simulink model "kundur_cvs_p2"  (R2025b)
settings: Solver=ode23t  StartTime=0.0  StopTime=0.5  MaxStep=0.005  RelTol=1e-3
values from neighbouring files (symbols this model uses):
  L_line_H = double(X_line_pu * Vbase^2 / Sbase / wn)    [build_kundur_cvs_p1.m]    (also in build_kundur_cvs_p2.m)
undefined symbols (not defined in the file or in its folder): D_1, D_2, D_3, D_4, delta0_1, delta0_2, delta0_3, delta0_4, M_1, M_2, M_3, M_4, Pe_scale, Pm_1, Pm_2, Pm_3, Pm_4, Vbase_const, wn_const
libraries: spsGroundLib x5, spsSeriesRLCBranchLib x5, spsControlledVoltageSourceLib x4, spsCurrentMeasurementLib x4, spsVoltageMeasurementLib x4, spsACVoltageSourceLib x1, spspowerguiLib x1
settings Model: Creator=27443  LastModifiedBy=27443

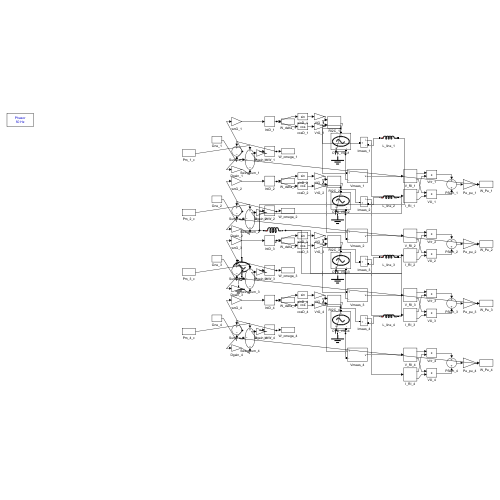
[thumbnail: Simulink's stored preview of the top-level diagram]
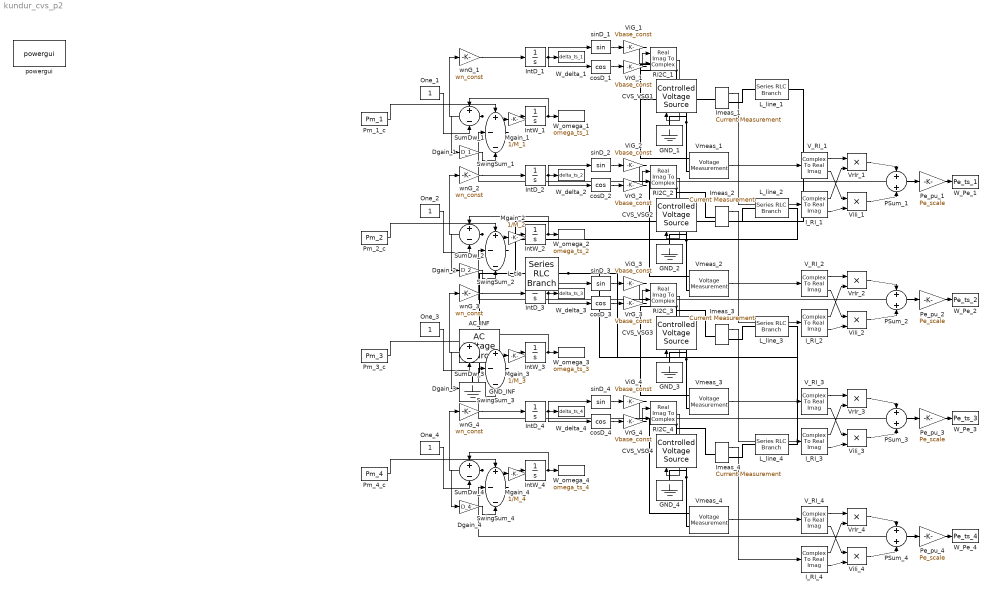
== system kundur_cvs_p2 ==
  AC_INF : spsACVoltageSourceLib/AC Voltage Source  Amplitude=230000  Phase=0  Frequency=50  SampleTime=0  Measurements=None  BusType=swing  Pref=10e3  Qref=0  Qmin=-inf  Qmax=+inf
  CVS_VSG{1..4} (4 alike) : spsControlledVoltageSourceLib/Controlled Voltage Source  Initialize=off  Source_Type=DC  Amplitude=230000  Phase=0  Frequency=0  Measurements=None
  Dgain_1 : Gain  Gain=D_1
  Dgain_2 : Gain  Gain=D_2
  Dgain_3 : Gain  Gain=D_3
  Dgain_4 : Gain  Gain=D_4
  GND_{1..4} (4 alike) : spsGroundLib/Ground  LConnTagsString=a
  GND_INF : spsGroundLib/Ground  LConnTagsString=a
  I_RI_{1..4} (4 alike) : ComplexToRealImag
  Imeas_{1..4} (4 alike) : spsCurrentMeasurementLib/Current Measurement  PhasorSimulation=on  OutputType=Complex  PSBequivalent=0
  IntD_1 : Integrator  InitialCondition=delta0_1
  IntD_2 : Integrator  InitialCondition=delta0_2
  IntD_3 : Integrator  InitialCondition=delta0_3
  IntD_4 : Integrator  InitialCondition=delta0_4
  IntW_{1..4} (4 alike) : Integrator  InitialCondition=1
  L_line_{1..4} (4 alike) : spsSeriesRLCBranchLib/Series RLC Branch  LConnTagsString=__new0  RConnTagsString=__new0  BranchType=L  Resistance=1  Inductance=L_line_H  SetiL0=off  InitialCurrent=0  Capacitance=1e-6  Setx0=off  InitialVoltage=0  Measurements=None
  L_tie : spsSeriesRLCBranchLib/Series RLC Branch  LConnTagsString=__new0  RConnTagsString=__new0  BranchType=L  Resistance=1  Inductance=0.50516  SetiL0=off  InitialCurrent=0  Capacitance=1e-6  Setx0=off  InitialVoltage=0  Measurements=None
  Mgain_1 : Gain  Gain=1/M_1
  Mgain_2 : Gain  Gain=1/M_2
  Mgain_3 : Gain  Gain=1/M_3
  Mgain_4 : Gain  Gain=1/M_4
  One_{1..4} (4 alike) : Constant
  PSum_{1..4} (4 alike) : Sum
  Pe_pu_{1..4} (4 alike) : Gain  Gain=Pe_scale
  Pm_1_c : Constant  Value=Pm_1
  Pm_2_c : Constant  Value=Pm_2
  Pm_3_c : Constant  Value=Pm_3
  Pm_4_c : Constant  Value=Pm_4
  RI2C_{1..4} (4 alike) : RealImagToComplex
  SumDw_{1..4} (4 alike) : Sum  Inputs=+-
  SwingSum_{1..4} (4 alike) : Sum  Inputs=+--
  V_RI_{1..4} (4 alike) : ComplexToRealImag
  ViG_{1..4} (4 alike) : Gain  Gain=Vbase_const
  ViIi_{1..4} (4 alike) : Product
  Vmeas_{1..4} (4 alike) : spsVoltageMeasurementLib/Voltage Measurement  PhasorSimulation=on  OutputType=Complex  PSBequivalent=0
  VrG_{1..4} (4 alike) : Gain  Gain=Vbase_const
  VrIr_{1..4} (4 alike) : Product
  W_Pe_1 : ToWorkspace  VariableName=Pe_ts_1  SaveFormat=Timeseries  SampleTime=-1
  W_Pe_2 : ToWorkspace  VariableName=Pe_ts_2  SaveFormat=Timeseries  SampleTime=-1
  W_Pe_3 : ToWorkspace  VariableName=Pe_ts_3  SaveFormat=Timeseries  SampleTime=-1
  W_Pe_4 : ToWorkspace  VariableName=Pe_ts_4  SaveFormat=Timeseries  SampleTime=-1
  W_delta_1 : ToWorkspace  VariableName=delta_ts_1  SaveFormat=Timeseries  SampleTime=-1
  W_delta_2 : ToWorkspace  VariableName=delta_ts_2  SaveFormat=Timeseries  SampleTime=-1
  W_delta_3 : ToWorkspace  VariableName=delta_ts_3  SaveFormat=Timeseries  SampleTime=-1
  W_delta_4 : ToWorkspace  VariableName=delta_ts_4  SaveFormat=Timeseries  SampleTime=-1
  W_omega_1 : ToWorkspace  VariableName=omega_ts_1  SaveFormat=Timeseries  SampleTime=-1
  W_omega_2 : ToWorkspace  VariableName=omega_ts_2  SaveFormat=Timeseries  SampleTime=-1
  W_omega_3 : ToWorkspace  VariableName=omega_ts_3  SaveFormat=Timeseries  SampleTime=-1
  W_omega_4 : ToWorkspace  VariableName=omega_ts_4  SaveFormat=Timeseries  SampleTime=-1
  cosD_{1..4} (4 alike) : Trigonometry  Operator=cos
  powergui : spspowerguiLib/powergui  Priority=1  SimulationMode=Phasor  SampleTime=50e-6  frequency=50  Iterations=50  frequencyindice=60  Pbase=100e6  ErrMax=1e-4  UnitsV=kV  UnitsW=MW  buscounter=0  FunctionMessages=off  echomessages=off  EnableUseOfTLC=off  CurrentSourceSwitches=off  DisableSnubberDevices=off  DisableRonSwitches=off  DisableVfSwitches=off  DisplayEquations=off  AutomaticDiscreteSolvers=off  SolverType=Tustin/Backward Euler (TBE)  Interpol=off  ExternalGateDelay=off  methode=off  Ts=100  x0status=blocks  SPID=on  SwTol=0  HookPort=off  NonlinearTolerance=1e-4  nMaxIteration=100  ContinueOnMaxIteration=off  RestoreLinks=warning  ResistiveCurrentMeasurement=off  Frange=[0:2:500]  Ylog=off  Xlog=on  ShowGrid=off  save=off  variable=ZData  structure=0  ZoomFFT=off  StartTime=0.0  cycles=1  DisplayStyle=1  fundamental=60  FreqAxis=off  MaxFrequency=1000  frequencyindicesteady=1  RmsSteady=1  display=off
  sinD_{1..4} (4 alike) : Trigonometry
  wnG_{1..4} (4 alike) : Gain  Gain=wn_const
  wires:
  Vmeas_1/1 -> V_RI_1/1
  Imeas_1/1 -> I_RI_1/1
  V_RI_1/1 -> VrIr_1/1
  I_RI_1/1 -> VrIr_1/2
  V_RI_1/2 -> ViIi_1/1
  I_RI_1/2 -> ViIi_1/2
  VrIr_1/1 -> PSum_1/1
  ViIi_1/1 -> PSum_1/2
  PSum_1/1 -> Pe_pu_1/1
  IntW_1/1 -> SumDw_1/1, W_omega_1/1
  One_1/1 -> SumDw_1/2
  SumDw_1/1 -> Dgain_1/1, wnG_1/1
  Pm_1_c/1 -> SwingSum_1/1
  Pe_pu_1/1 -> SwingSum_1/2, W_Pe_1/1
  Dgain_1/1 -> SwingSum_1/3
  SwingSum_1/1 -> Mgain_1/1
  Mgain_1/1 -> IntW_1/1
  wnG_1/1 -> IntD_1/1
  IntD_1/1 -> cosD_1/1, sinD_1/1, W_delta_1/1
  cosD_1/1 -> VrG_1/1
  sinD_1/1 -> ViG_1/1
  VrG_1/1 -> RI2C_1/1
  ViG_1/1 -> RI2C_1/2
  RI2C_1/1 -> CVS_VSG1/1
  Vmeas_2/1 -> V_RI_2/1
  Imeas_2/1 -> I_RI_2/1
  V_RI_2/1 -> VrIr_2/1
  I_RI_2/1 -> VrIr_2/2
  V_RI_2/2 -> ViIi_2/1
  I_RI_2/2 -> ViIi_2/2
  VrIr_2/1 -> PSum_2/1
  ViIi_2/1 -> PSum_2/2
  PSum_2/1 -> Pe_pu_2/1
  IntW_2/1 -> SumDw_2/1, W_omega_2/1
  One_2/1 -> SumDw_2/2
  SumDw_2/1 -> Dgain_2/1, wnG_2/1
  Pm_2_c/1 -> SwingSum_2/1
  Pe_pu_2/1 -> SwingSum_2/2, W_Pe_2/1
  Dgain_2/1 -> SwingSum_2/3
  SwingSum_2/1 -> Mgain_2/1
  Mgain_2/1 -> IntW_2/1
  wnG_2/1 -> IntD_2/1
  IntD_2/1 -> cosD_2/1, sinD_2/1, W_delta_2/1
  cosD_2/1 -> VrG_2/1
  sinD_2/1 -> ViG_2/1
  VrG_2/1 -> RI2C_2/1
  ViG_2/1 -> RI2C_2/2
  RI2C_2/1 -> CVS_VSG2/1
  Vmeas_3/1 -> V_RI_3/1
  Imeas_3/1 -> I_RI_3/1
  V_RI_3/1 -> VrIr_3/1
  I_RI_3/1 -> VrIr_3/2
  V_RI_3/2 -> ViIi_3/1
  I_RI_3/2 -> ViIi_3/2
  VrIr_3/1 -> PSum_3/1
  ViIi_3/1 -> PSum_3/2
  PSum_3/1 -> Pe_pu_3/1
  IntW_3/1 -> SumDw_3/1, W_omega_3/1
  One_3/1 -> SumDw_3/2
  SumDw_3/1 -> Dgain_3/1, wnG_3/1
  Pm_3_c/1 -> SwingSum_3/1
  Pe_pu_3/1 -> SwingSum_3/2, W_Pe_3/1
  Dgain_3/1 -> SwingSum_3/3
  SwingSum_3/1 -> Mgain_3/1
  Mgain_3/1 -> IntW_3/1
  wnG_3/1 -> IntD_3/1
  IntD_3/1 -> cosD_3/1, sinD_3/1, W_delta_3/1
  cosD_3/1 -> VrG_3/1
  sinD_3/1 -> ViG_3/1
  VrG_3/1 -> RI2C_3/1
  ViG_3/1 -> RI2C_3/2
  RI2C_3/1 -> CVS_VSG3/1
  Vmeas_4/1 -> V_RI_4/1
  Imeas_4/1 -> I_RI_4/1
  V_RI_4/1 -> VrIr_4/1
  I_RI_4/1 -> VrIr_4/2
  V_RI_4/2 -> ViIi_4/1
  I_RI_4/2 -> ViIi_4/2
  VrIr_4/1 -> PSum_4/1
  ViIi_4/1 -> PSum_4/2
  PSum_4/1 -> Pe_pu_4/1
  IntW_4/1 -> SumDw_4/1, W_omega_4/1
  One_4/1 -> SumDw_4/2
  SumDw_4/1 -> Dgain_4/1, wnG_4/1
  Pm_4_c/1 -> SwingSum_4/1
  Pe_pu_4/1 -> SwingSum_4/2, W_Pe_4/1
  Dgain_4/1 -> SwingSum_4/3
  SwingSum_4/1 -> Mgain_4/1
  Mgain_4/1 -> IntW_4/1
  wnG_4/1 -> IntD_4/1
  IntD_4/1 -> cosD_4/1, sinD_4/1, W_delta_4/1
  cosD_4/1 -> VrG_4/1
  sinD_4/1 -> ViG_4/1
  VrG_4/1 -> RI2C_4/1
  ViG_4/1 -> RI2C_4/2
  RI2C_4/1 -> CVS_VSG4/1
  connections:
  AC_INF/RConn1 -- L_line_1/RConn1 -- L_tie/LConn1 -- L_line_2/RConn1
  AC_INF/LConn1 -- GND_INF/LConn1
  Imeas_1/LConn1 -- CVS_VSG1/RConn1 -- Vmeas_1/LConn1
  Imeas_1/RConn1 -- L_line_1/LConn1
  GND_1/LConn1 -- CVS_VSG1/LConn1 -- Vmeas_1/LConn2
  Imeas_2/LConn1 -- CVS_VSG2/RConn1 -- Vmeas_2/LConn1
  Imeas_2/RConn1 -- L_line_2/LConn1
  GND_2/LConn1 -- CVS_VSG2/LConn1 -- Vmeas_2/LConn2
  Imeas_3/LConn1 -- CVS_VSG3/RConn1 -- Vmeas_3/LConn1
  Imeas_3/RConn1 -- L_line_3/LConn1
  GND_3/LConn1 -- CVS_VSG3/LConn1 -- Vmeas_3/LConn2
  L_tie/RConn1 -- L_line_3/RConn1 -- L_line_4/RConn1
  Imeas_4/LConn1 -- CVS_VSG4/RConn1 -- Vmeas_4/LConn1
  Imeas_4/RConn1 -- L_line_4/LConn1
  GND_4/LConn1 -- CVS_VSG4/LConn1 -- Vmeas_4/LConn2
